simulink model "tracker"  (R2020a)
settings: Solver=VariableStepAuto  StartTime=0.0  StopTime=simulation_time  RelTol=1e-3
values from neighbouring files (symbols this model uses):
  costas_pll_arctan_nstage = 8    [tracker_hw_init.m]
  costas_pll_arctan_point = 16    [tracker_hw_init.m]
  costas_pll_arctan_width = 32    [tracker_hw_init.m]
  DDS_ch_pinc = fc.*(2^(DDS_phase_width)/fs)    [tracker_hw_init.m]
  fs = 120e6    (= 120000000)    [tracker_hw_init.m]
  normalized_EML_power_cordic_nstage = 11    [tracker_hw_init.m]
  normalized_EML_power_cordic_point = 32    [tracker_hw_init.m]
  normalized_EML_power_cordic_width = 32    [tracker_hw_init.m]
  ts = 1/fs    (= 8.33333333333e-09)    [tracker_hw_init.m]
undefined symbols (not defined in the file or in its folder): cacode, i
libraries: xbsIndex_r4 x1873
(part 1 of 14)
settings Model: Creator=User  LastModifiedBy=sysgen

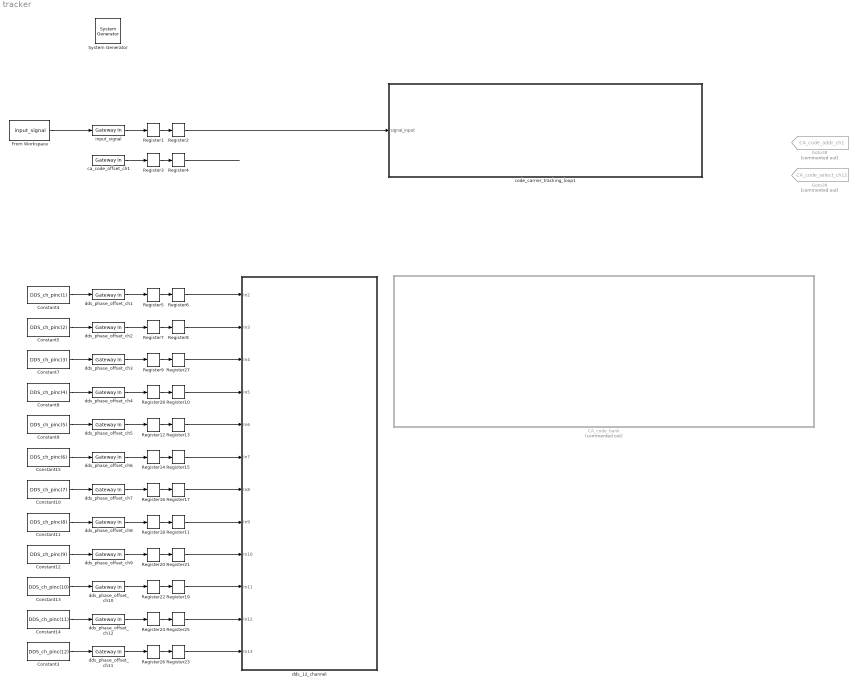
== system tracker ==
  " System Generator" : xbsIndex_r4/ System Generator  Tag=genX  xilinxfamily=zynquplus  part=xczu7ev  speed=-1-i  package=fbvb900  synthesis_tool=Vivado  clock_wrapper=Clock Enables  directory=./netlist  proj_type=Vivado  Synth_file=Vivado Synthesis Defaults  Impl_file=Vivado Implementation Defaults  testbench=off  simulink_period=ts  sysclk_period=ts*1e9  dcm_input_clock_period=10  incr_netlist=off  trim_vbits=Everywhere in SubSystem  dbl_ovrd=According to Block Masks  core_generation=According to Block Masks  run_coregen=off  deprecated_control=off  eval_field=0  block_type=sysgen
  CA_code_bank : Subsystem  Commented=on
  Constant10 : Constant  Value=DDS_ch_pinc(7)
  Constant11 : Constant  Value=DDS_ch_pinc(8)
  Constant12 : Constant  Value=DDS_ch_pinc(9)
  Constant13 : Constant  Value=DDS_ch_pinc(10)
  Constant14 : Constant  Value=DDS_ch_pinc(11)
  Constant15 : Constant  Value=DDS_ch_pinc(6)
  Constant3 : Constant  Value=DDS_ch_pinc(12)
  Constant4 : Constant  Value=DDS_ch_pinc(1)
  Constant5 : Constant  Value=DDS_ch_pinc(2)
  Constant7 : Constant  Value=DDS_ch_pinc(3)
  Constant8 : Constant  Value=DDS_ch_pinc(4)
  Constant9 : Constant  Value=DDS_ch_pinc(5)
  From Workspace : FromWorkspace  VariableName=input_signal  SampleTime=-1  OutputAfterFinalValue=Setting to zero
  Goto38 : Goto  Commented=on  GotoTag=CA_code_addr_ch1  TagVisibility=global
  Goto39 : Goto  Commented=on  GotoTag=CA_code_select_ch12  TagVisibility=global
  Register{1..28} (28 alike) : xbsIndex_r4/Register  init=0  rst=off  en=off  dbl_ovrd=off  block_type=register
  ca_code_offset_ch1 : xbsIndex_r4/Gateway In  gui_display_data_type=Fixed-point  arith_type=Unsigned  n_bits=DDS_phase_width  bin_pt=DDS_phase_width  preci_type=Single  exp_width=8  frac_width=24  rows=1  columns=1  quantization="Round  (unbiased: +/- Inf)"  overflow=Saturate  period=12*ts  UseAsADC=off  ADCChannel='1'  interface=None  automatic_assignment=on  address_offset=hex2dec('00')  intf_name=''  intf_description=''  default_value=0  timing_constraint=None  locs_specified=off  LOCs={}  io_standard={}  inherit_from_input=off  hdl_port=on  dbl_ovrd=off  block_type=gatewayin
  code_carrier_tracking_loop1 : Subsystem
  dds_12_channel : Subsystem
  dds_phase_offset_ch{1..12} (12 alike) : xbsIndex_r4/Gateway In  gui_display_data_type=Fixed-point  arith_type=Unsigned  n_bits=DDS_phase_width  bin_pt=DDS_phase_width  preci_type=Single  exp_width=8  frac_width=24  rows=1  columns=1  quantization="Round  (unbiased: +/- Inf)"  overflow=Saturate  period=ts  UseAsADC=off  ADCChannel='1'  interface=None  automatic_assignment=on  address_offset=hex2dec('00')  intf_name=''  intf_description=''  default_value=0  timing_constraint=None  locs_specified=off  LOCs={}  io_standard={}  inherit_from_input=off  hdl_port=on  dbl_ovrd=off  block_type=gatewayin
  input_signal : xbsIndex_r4/Gateway In  gui_display_data_type=Fixed-point  arith_type="Signed  (2's comp)"  n_bits=input_signal_width  bin_pt=input_signal_binary_point  preci_type=Single  exp_width=8  frac_width=24  rows=1  columns=1  quantization="Round  (unbiased: +/- Inf)"  overflow=Saturate  period=12*ts  UseAsADC=off  ADCChannel='1'  interface=None  automatic_assignment=on  address_offset=hex2dec('00')  intf_name=''  intf_description=''  default_value=0  timing_constraint=None  locs_specified=off  LOCs={}  io_standard={}  inherit_from_input=off  hdl_port=on  dbl_ovrd=off  block_type=gatewayin
  wires:
  dds_phase_offset_ch9/1 -> Register20/1
  Constant9/1 -> dds_phase_offset_ch5/1
  Constant4/1 -> dds_phase_offset_ch1/1
  Constant10/1 -> dds_phase_offset_ch7/1
  Constant11/1 -> dds_phase_offset_ch8/1
  Constant13/1 -> dds_phase_offset_ch10/1
  Constant3/1 -> dds_phase_offset_ch11/1
  dds_phase_offset_ch12/1 -> Register24/1
  Register22/1 -> Register19/1
  dds_phase_offset_ch6/1 -> Register14/1
  Register26/1 -> Register23/1
  dds_phase_offset_ch7/1 -> Register16/1
  Register20/1 -> Register21/1
  Constant12/1 -> dds_phase_offset_ch9/1
  Constant8/1 -> dds_phase_offset_ch4/1
  dds_phase_offset_ch11/1 -> Register26/1
  Constant5/1 -> dds_phase_offset_ch2/1
  Constant7/1 -> dds_phase_offset_ch3/1
  Constant15/1 -> dds_phase_offset_ch6/1
  dds_phase_offset_ch5/1 -> Register12/1
  Register24/1 -> Register25/1
  Constant14/1 -> dds_phase_offset_ch12/1
  dds_phase_offset_ch8/1 -> Register18/1
  Register5/1 -> Register6/1
  Register28/1 -> Register10/1
  dds_phase_offset_ch2/1 -> Register7/1
  Register18/1 -> Register11/1
  Register12/1 -> Register13/1
  dds_phase_offset_ch4/1 -> Register28/1
  Register16/1 -> Register17/1
  dds_phase_offset_ch3/1 -> Register9/1
  Register7/1 -> Register8/1
  Register9/1 -> Register27/1
  dds_phase_offset_ch1/1 -> Register5/1
  dds_phase_offset_ch10/1 -> Register22/1
  Register14/1 -> Register15/1
  Register6/1 -> dds_12_channel/1(In2)
  Register8/1 -> dds_12_channel/2(In3)
  Register27/1 -> dds_12_channel/3(In4)
  Register10/1 -> dds_12_channel/4(In5)
  Register13/1 -> dds_12_channel/5(In6)
  Register15/1 -> dds_12_channel/6(In7)
  Register17/1 -> dds_12_channel/7(In8)
  Register11/1 -> dds_12_channel/8(In9)
  Register21/1 -> dds_12_channel/9(In10)
  Register19/1 -> dds_12_channel/10(In11)
  Register25/1 -> dds_12_channel/11(In12)
  Register23/1 -> dds_12_channel/12(In13)
  input_signal/1 -> Register1/1
  Register1/1 -> Register2/1
  Register2/1 -> code_carrier_tracking_loop1/1(signal_input)
  From Workspace/1 -> input_signal/1
  Register4/1 -> ?
  ca_code_offset_ch1/1 -> Register3/1
  Register3/1 -> Register4/1

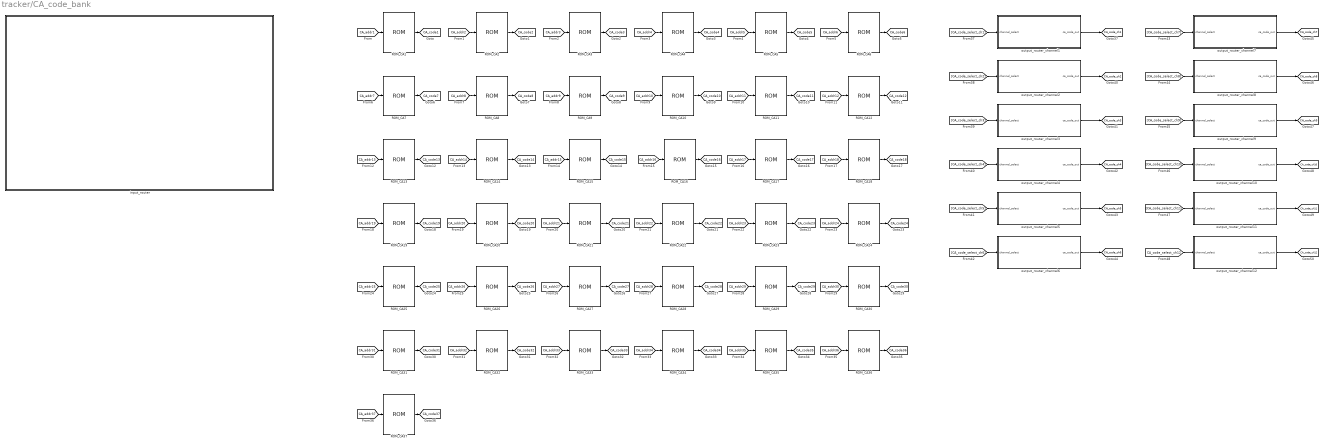
== system tracker/CA_code_bank ==
  ROM_CA1 : xbsIndex_r4/ROM  depth=1023  initVector=cacode(1,1)  distributed_mem=Distributed memory  rst=off  init_reg=0  en=off  latency=1  gui_display_data_type=Boolean  arith_type=Boolean  n_bits=16  bin_pt=14  preci_type=Single  exp_width=8  frac_width=24  optimize=Area  use_rpm=on  dbl_ovrd=off  simulation_type=fast_sim  block_type=sprom
  ROM_CA10 : xbsIndex_r4/ROM  depth=1023  initVector=cacode(10,1)  distributed_mem=Distributed memory  rst=off  init_reg=0  en=off  latency=1  gui_display_data_type=Boolean  arith_type=Boolean  n_bits=16  bin_pt=14  preci_type=Single  exp_width=8  frac_width=24  optimize=Area  use_rpm=on  dbl_ovrd=off  simulation_type=fast_sim  block_type=sprom
  ROM_CA11 : xbsIndex_r4/ROM  depth=1023  initVector=cacode(11,1)  distributed_mem=Distributed memory  rst=off  init_reg=0  en=off  latency=1  gui_display_data_type=Boolean  arith_type=Boolean  n_bits=16  bin_pt=14  preci_type=Single  exp_width=8  frac_width=24  optimize=Area  use_rpm=on  dbl_ovrd=off  simulation_type=fast_sim  block_type=sprom
  ROM_CA12 : xbsIndex_r4/ROM  depth=1023  initVector=cacode(12,1)  distributed_mem=Distributed memory  rst=off  init_reg=0  en=off  latency=1  gui_display_data_type=Boolean  arith_type=Boolean  n_bits=16  bin_pt=14  preci_type=Single  exp_width=8  frac_width=24  optimize=Area  use_rpm=on  dbl_ovrd=off  simulation_type=fast_sim  block_type=sprom
  ROM_CA13 : xbsIndex_r4/ROM  depth=1023  initVector=cacode(13,1)  distributed_mem=Distributed memory  rst=off  init_reg=0  en=off  latency=1  gui_display_data_type=Boolean  arith_type=Boolean  n_bits=16  bin_pt=14  preci_type=Single  exp_width=8  frac_width=24  optimize=Area  use_rpm=on  dbl_ovrd=off  simulation_type=fast_sim  block_type=sprom
  ROM_CA14 : xbsIndex_r4/ROM  depth=1023  initVector=cacode(14,1)  distributed_mem=Distributed memory  rst=off  init_reg=0  en=off  latency=1  gui_display_data_type=Boolean  arith_type=Boolean  n_bits=16  bin_pt=14  preci_type=Single  exp_width=8  frac_width=24  optimize=Area  use_rpm=on  dbl_ovrd=off  simulation_type=fast_sim  block_type=sprom
  ROM_CA15 : xbsIndex_r4/ROM  depth=1023  initVector=cacode(15,1)  distributed_mem=Distributed memory  rst=off  init_reg=0  en=off  latency=1  gui_display_data_type=Boolean  arith_type=Boolean  n_bits=16  bin_pt=14  preci_type=Single  exp_width=8  frac_width=24  optimize=Area  use_rpm=on  dbl_ovrd=off  simulation_type=fast_sim  block_type=sprom
  ROM_CA16 : xbsIndex_r4/ROM  depth=1023  initVector=cacode(16,1)  distributed_mem=Distributed memory  rst=off  init_reg=0  en=off  latency=1  gui_display_data_type=Boolean  arith_type=Boolean  n_bits=16  bin_pt=14  preci_type=Single  exp_width=8  frac_width=24  optimize=Area  use_rpm=on  dbl_ovrd=off  simulation_type=fast_sim  block_type=sprom
  ROM_CA17 : xbsIndex_r4/ROM  depth=1023  initVector=cacode(17,1)  distributed_mem=Distributed memory  rst=off  init_reg=0  en=off  latency=1  gui_display_data_type=Boolean  arith_type=Boolean  n_bits=16  bin_pt=14  preci_type=Single  exp_width=8  frac_width=24  optimize=Area  use_rpm=on  dbl_ovrd=off  simulation_type=fast_sim  block_type=sprom
  ROM_CA18 : xbsIndex_r4/ROM  depth=1023  initVector=cacode(18,1)  distributed_mem=Distributed memory  rst=off  init_reg=0  en=off  latency=1  gui_display_data_type=Boolean  arith_type=Boolean  n_bits=16  bin_pt=14  preci_type=Single  exp_width=8  frac_width=24  optimize=Area  use_rpm=on  dbl_ovrd=off  simulation_type=fast_sim  block_type=sprom
  ROM_CA19 : xbsIndex_r4/ROM  depth=1023  initVector=cacode(19,1)  distributed_mem=Distributed memory  rst=off  init_reg=0  en=off  latency=1  gui_display_data_type=Boolean  arith_type=Boolean  n_bits=16  bin_pt=14  preci_type=Single  exp_width=8  frac_width=24  optimize=Area  use_rpm=on  dbl_ovrd=off  simulation_type=fast_sim  block_type=sprom
  ROM_CA2 : xbsIndex_r4/ROM  depth=1023  initVector=cacode(2,1)  distributed_mem=Distributed memory  rst=off  init_reg=0  en=off  latency=1  gui_display_data_type=Boolean  arith_type=Boolean  n_bits=16  bin_pt=14  preci_type=Single  exp_width=8  frac_width=24  optimize=Area  use_rpm=on  dbl_ovrd=off  simulation_type=fast_sim  block_type=sprom
  ROM_CA20 : xbsIndex_r4/ROM  depth=1023  initVector=cacode(20,1)  distributed_mem=Distributed memory  rst=off  init_reg=0  en=off  latency=1  gui_display_data_type=Boolean  arith_type=Boolean  n_bits=16  bin_pt=14  preci_type=Single  exp_width=8  frac_width=24  optimize=Area  use_rpm=on  dbl_ovrd=off  simulation_type=fast_sim  block_type=sprom
  ROM_CA21 : xbsIndex_r4/ROM  depth=1023  initVector=cacode(21,1)  distributed_mem=Distributed memory  rst=off  init_reg=0  en=off  latency=1  gui_display_data_type=Boolean  arith_type=Boolean  n_bits=16  bin_pt=14  preci_type=Single  exp_width=8  frac_width=24  optimize=Area  use_rpm=on  dbl_ovrd=off  simulation_type=fast_sim  block_type=sprom
  ROM_CA22 : xbsIndex_r4/ROM  depth=1023  initVector=cacode(22,1)  distributed_mem=Distributed memory  rst=off  init_reg=0  en=off  latency=1  gui_display_data_type=Boolean  arith_type=Boolean  n_bits=16  bin_pt=14  preci_type=Single  exp_width=8  frac_width=24  optimize=Area  use_rpm=on  dbl_ovrd=off  simulation_type=fast_sim  block_type=sprom
  ROM_CA23 : xbsIndex_r4/ROM  depth=1023  initVector=cacode(23,1)  distributed_mem=Distributed memory  rst=off  init_reg=0  en=off  latency=1  gui_display_data_type=Boolean  arith_type=Boolean  n_bits=16  bin_pt=14  preci_type=Single  exp_width=8  frac_width=24  optimize=Area  use_rpm=on  dbl_ovrd=off  simulation_type=fast_sim  block_type=sprom
  ROM_CA24 : xbsIndex_r4/ROM  depth=1023  initVector=cacode(24,1)  distributed_mem=Distributed memory  rst=off  init_reg=0  en=off  latency=1  gui_display_data_type=Boolean  arith_type=Boolean  n_bits=16  bin_pt=14  preci_type=Single  exp_width=8  frac_width=24  optimize=Area  use_rpm=on  dbl_ovrd=off  simulation_type=fast_sim  block_type=sprom
  ROM_CA25 : xbsIndex_r4/ROM  depth=1023  initVector=cacode(25,1)  distributed_mem=Distributed memory  rst=off  init_reg=0  en=off  latency=1  gui_display_data_type=Boolean  arith_type=Boolean  n_bits=16  bin_pt=14  preci_type=Single  exp_width=8  frac_width=24  optimize=Area  use_rpm=on  dbl_ovrd=off  simulation_type=fast_sim  block_type=sprom
  ROM_CA26 : xbsIndex_r4/ROM  depth=1023  initVector=cacode(26,1)  distributed_mem=Distributed memory  rst=off  init_reg=0  en=off  latency=1  gui_display_data_type=Boolean  arith_type=Boolean  n_bits=16  bin_pt=14  preci_type=Single  exp_width=8  frac_width=24  optimize=Area  use_rpm=on  dbl_ovrd=off  simulation_type=fast_sim  block_type=sprom
  ROM_CA27 : xbsIndex_r4/ROM  depth=1023  initVector=cacode(27,1)  distributed_mem=Distributed memory  rst=off  init_reg=0  en=off  latency=1  gui_display_data_type=Boolean  arith_type=Boolean  n_bits=16  bin_pt=14  preci_type=Single  exp_width=8  frac_width=24  optimize=Area  use_rpm=on  dbl_ovrd=off  simulation_type=fast_sim  block_type=sprom
  ROM_CA28 : xbsIndex_r4/ROM  depth=1023  initVector=cacode(28,1)  distributed_mem=Distributed memory  rst=off  init_reg=0  en=off  latency=1  gui_display_data_type=Boolean  arith_type=Boolean  n_bits=16  bin_pt=14  preci_type=Single  exp_width=8  frac_width=24  optimize=Area  use_rpm=on  dbl_ovrd=off  simulation_type=fast_sim  block_type=sprom
  ROM_CA29 : xbsIndex_r4/ROM  depth=1023  initVector=cacode(29,1)  distributed_mem=Distributed memory  rst=off  init_reg=0  en=off  latency=1  gui_display_data_type=Boolean  arith_type=Boolean  n_bits=16  bin_pt=14  preci_type=Single  exp_width=8  frac_width=24  optimize=Area  use_rpm=on  dbl_ovrd=off  simulation_type=fast_sim  block_type=sprom
  ROM_CA3 : xbsIndex_r4/ROM  depth=1023  initVector=cacode(3,1)  distributed_mem=Distributed memory  rst=off  init_reg=0  en=off  latency=1  gui_display_data_type=Boolean  arith_type=Boolean  n_bits=16  bin_pt=14  preci_type=Single  exp_width=8  frac_width=24  optimize=Area  use_rpm=on  dbl_ovrd=off  simulation_type=fast_sim  block_type=sprom
  ROM_CA30 : xbsIndex_r4/ROM  depth=1023  initVector=cacode(30,1)  distributed_mem=Distributed memory  rst=off  init_reg=0  en=off  latency=1  gui_display_data_type=Boolean  arith_type=Boolean  n_bits=16  bin_pt=14  preci_type=Single  exp_width=8  frac_width=24  optimize=Area  use_rpm=on  dbl_ovrd=off  simulation_type=fast_sim  block_type=sprom
  ROM_CA31 : xbsIndex_r4/ROM  depth=1023  initVector=cacode(31,1)  distributed_mem=Distributed memory  rst=off  init_reg=0  en=off  latency=1  gui_display_data_type=Boolean  arith_type=Boolean  n_bits=16  bin_pt=14  preci_type=Single  exp_width=8  frac_width=24  optimize=Area  use_rpm=on  dbl_ovrd=off  simulation_type=fast_sim  block_type=sprom
  ROM_CA32 : xbsIndex_r4/ROM  depth=1023  initVector=cacode(32,1)  distributed_mem=Distributed memory  rst=off  init_reg=0  en=off  latency=1  gui_display_data_type=Boolean  arith_type=Boolean  n_bits=16  bin_pt=14  preci_type=Single  exp_width=8  frac_width=24  optimize=Area  use_rpm=on  dbl_ovrd=off  simulation_type=fast_sim  block_type=sprom
  ROM_CA33 : xbsIndex_r4/ROM  depth=1023  initVector=cacode(33,1)  distributed_mem=Distributed memory  rst=off  init_reg=0  en=off  latency=1  gui_display_data_type=Boolean  arith_type=Boolean  n_bits=16  bin_pt=14  preci_type=Single  exp_width=8  frac_width=24  optimize=Area  use_rpm=on  dbl_ovrd=off  simulation_type=fast_sim  block_type=sprom
  ROM_CA34 : xbsIndex_r4/ROM  depth=1023  initVector=cacode(34,1)  distributed_mem=Distributed memory  rst=off  init_reg=0  en=off  latency=1  gui_display_data_type=Boolean  arith_type=Boolean  n_bits=16  bin_pt=14  preci_type=Single  exp_width=8  frac_width=24  optimize=Area  use_rpm=on  dbl_ovrd=off  simulation_type=fast_sim  block_type=sprom
  ROM_CA35 : xbsIndex_r4/ROM  depth=1023  initVector=cacode(35,1)  distributed_mem=Distributed memory  rst=off  init_reg=0  en=off  latency=1  gui_display_data_type=Boolean  arith_type=Boolean  n_bits=16  bin_pt=14  preci_type=Single  exp_width=8  frac_width=24  optimize=Area  use_rpm=on  dbl_ovrd=off  simulation_type=fast_sim  block_type=sprom
  ROM_CA36 : xbsIndex_r4/ROM  depth=1023  initVector=cacode(36,1)  distributed_mem=Distributed memory  rst=off  init_reg=0  en=off  latency=1  gui_display_data_type=Boolean  arith_type=Boolean  n_bits=16  bin_pt=14  preci_type=Single  exp_width=8  frac_width=24  optimize=Area  use_rpm=on  dbl_ovrd=off  simulation_type=fast_sim  block_type=sprom
  ROM_CA37 : xbsIndex_r4/ROM  depth=1023  initVector=cacode(37,1)  distributed_mem=Distributed memory  rst=off  init_reg=0  en=off  latency=1  gui_display_data_type=Boolean  arith_type=Boolean  n_bits=16  bin_pt=14  preci_type=Single  exp_width=8  frac_width=24  optimize=Area  use_rpm=on  dbl_ovrd=off  simulation_type=fast_sim  block_type=sprom
  ROM_CA4 : xbsIndex_r4/ROM  depth=1023  initVector=cacode(4,1)  distributed_mem=Distributed memory  rst=off  init_reg=0  en=off  latency=1  gui_display_data_type=Boolean  arith_type=Boolean  n_bits=16  bin_pt=14  preci_type=Single  exp_width=8  frac_width=24  optimize=Area  use_rpm=on  dbl_ovrd=off  simulation_type=fast_sim  block_type=sprom
  ROM_CA5 : xbsIndex_r4/ROM  depth=1023  initVector=cacode(5,1)  distributed_mem=Distributed memory  rst=off  init_reg=0  en=off  latency=1  gui_display_data_type=Boolean  arith_type=Boolean  n_bits=16  bin_pt=14  preci_type=Single  exp_width=8  frac_width=24  optimize=Area  use_rpm=on  dbl_ovrd=off  simulation_type=fast_sim  block_type=sprom
  ROM_CA6 : xbsIndex_r4/ROM  depth=1023  initVector=cacode(6,1)  distributed_mem=Distributed memory  rst=off  init_reg=0  en=off  latency=1  gui_display_data_type=Boolean  arith_type=Boolean  n_bits=16  bin_pt=14  preci_type=Single  exp_width=8  frac_width=24  optimize=Area  use_rpm=on  dbl_ovrd=off  simulation_type=fast_sim  block_type=sprom
  ROM_CA7 : xbsIndex_r4/ROM  depth=1023  initVector=cacode(7,1)  distributed_mem=Distributed memory  rst=off  init_reg=0  en=off  latency=1  gui_display_data_type=Boolean  arith_type=Boolean  n_bits=16  bin_pt=14  preci_type=Single  exp_width=8  frac_width=24  optimize=Area  use_rpm=on  dbl_ovrd=off  simulation_type=fast_sim  block_type=sprom
  ROM_CA8 : xbsIndex_r4/ROM  depth=1023  initVector=cacode(8,1)  distributed_mem=Distributed memory  rst=off  init_reg=0  en=off  latency=1  gui_display_data_type=Boolean  arith_type=Boolean  n_bits=16  bin_pt=14  preci_type=Single  exp_width=8  frac_width=24  optimize=Area  use_rpm=on  dbl_ovrd=off  simulation_type=fast_sim  block_type=sprom
  ROM_CA9 : xbsIndex_r4/ROM  depth=1023  initVector=cacode(9,1)  distributed_mem=Distributed memory  rst=off  init_reg=0  en=off  latency=1  gui_display_data_type=Boolean  arith_type=Boolean  n_bits=16  bin_pt=14  preci_type=Single  exp_width=8  frac_width=24  optimize=Area  use_rpm=on  dbl_ovrd=off  simulation_type=fast_sim  block_type=sprom
  input_router : Subsystem
  output_router_channel1 : Subsystem
  output_router_channel10 : Subsystem
  output_router_channel11 : Subsystem
  output_router_channel12 : Subsystem
  output_router_channel2 : Subsystem
  output_router_channel3 : Subsystem
  output_router_channel4 : Subsystem
  output_router_channel5 : Subsystem
  output_router_channel6 : Subsystem
  output_router_channel7 : Subsystem
  output_router_channel8 : Subsystem
  output_router_channel9 : Subsystem
  tag scope: CA_code10=global, CA_code11=global, CA_code12=global, CA_code13=global, CA_code14=global, CA_code15=global, CA_code16=global, CA_code17=global, CA_code18=global, CA_code19=global, CA_code1=global, CA_code20=global, CA_code21=global, CA_code22=global, CA_code23=global, CA_code24=global, CA_code25=global, CA_code26=global, CA_code27=global, CA_code28=global, CA_code29=global, CA_code2=global, CA_code30=global, CA_code31=global, CA_code32=global, CA_code33=global, CA_code34=global, CA_code35=global, CA_code36=global, CA_code37=global, CA_code3=global, CA_code4=global, CA_code5=global, CA_code6=global, CA_code7=global, CA_code8=global, CA_code9=global, CA_code_ch10=global, CA_code_ch11=global, CA_code_ch12=global, CA_code_ch1=global, CA_code_ch2=global, CA_code_ch3=global, CA_code_ch4=global, CA_code_ch5=global, CA_code_ch6=global, CA_code_ch7=global, CA_code_ch8=global, CA_code_ch9=global
  wires:
  ROM_CA1/1 -> [CA_code1]
  ROM_CA2/1 -> [CA_code2]
  ROM_CA3/1 -> [CA_code3]
  ROM_CA4/1 -> [CA_code4]
  ROM_CA5/1 -> [CA_code5]
  ROM_CA6/1 -> [CA_code6]
  ROM_CA7/1 -> [CA_code7]
  ROM_CA8/1 -> [CA_code8]
  ROM_CA9/1 -> [CA_code9]
  ROM_CA10/1 -> [CA_code10]
  ROM_CA11/1 -> [CA_code11]
  ROM_CA12/1 -> [CA_code12]
  ROM_CA13/1 -> [CA_code13]
  ROM_CA14/1 -> [CA_code14]
  ROM_CA15/1 -> [CA_code15]
  ROM_CA16/1 -> [CA_code16]
  ROM_CA17/1 -> [CA_code17]
  ROM_CA18/1 -> [CA_code18]
  ROM_CA19/1 -> [CA_code19]
  [CA_addr1] -> ROM_CA1/1
  [CA_addr2] -> ROM_CA2/1
  [CA_addr3] -> ROM_CA3/1
  [CA_addr4] -> ROM_CA4/1
  [CA_addr5] -> ROM_CA5/1
  [CA_addr6] -> ROM_CA6/1
  [CA_addr7] -> ROM_CA7/1
  [CA_addr8] -> ROM_CA8/1
  [CA_addr9] -> ROM_CA9/1
  [CA_addr10] -> ROM_CA10/1
  [CA_addr11] -> ROM_CA11/1
  [CA_addr12] -> ROM_CA12/1
  [CA_addr13] -> ROM_CA13/1
  [CA_addr14] -> ROM_CA14/1
  [CA_addr15] -> ROM_CA15/1
  [CA_addr16] -> ROM_CA16/1
  [CA_addr17] -> ROM_CA17/1
  [CA_addr18] -> ROM_CA18/1
  [CA_addr19] -> ROM_CA19/1
  [CA_addr20] -> ROM_CA20/1
  ROM_CA20/1 -> [CA_code20]
  [CA_addr21] -> ROM_CA21/1
  ROM_CA21/1 -> [CA_code21]
  [CA_addr22] -> ROM_CA22/1
  ROM_CA22/1 -> [CA_code22]
  [CA_addr23] -> ROM_CA23/1
  ROM_CA23/1 -> [CA_code23]
  [CA_addr24] -> ROM_CA24/1
  ROM_CA24/1 -> [CA_code24]
  [CA_addr25] -> ROM_CA25/1
  ROM_CA25/1 -> [CA_code25]
  [CA_addr26] -> ROM_CA26/1
  ROM_CA26/1 -> [CA_code26]
  [CA_addr27] -> ROM_CA27/1
  ROM_CA27/1 -> [CA_code27]
  ROM_CA28/1 -> [CA_code28]
  [CA_addr28] -> ROM_CA28/1
  ROM_CA29/1 -> [CA_code29]
  [CA_addr29] -> ROM_CA29/1
  [CA_addr30] -> ROM_CA30/1
  ROM_CA30/1 -> [CA_code30]
  [CA_addr31] -> ROM_CA31/1
  ROM_CA31/1 -> [CA_code31]
  [CA_addr32] -> ROM_CA32/1
  ROM_CA32/1 -> [CA_code32]
  [CA_addr33] -> ROM_CA33/1
  ROM_CA33/1 -> [CA_code33]
  [CA_addr34] -> ROM_CA34/1
  ROM_CA34/1 -> [CA_code34]
  [CA_addr35] -> ROM_CA35/1
  ROM_CA35/1 -> [CA_code35]
  [CA_addr36] -> ROM_CA36/1
  ROM_CA36/1 -> [CA_code36]
  ROM_CA37/1 -> [CA_code37]
  [CA_addr37] -> ROM_CA37/1
  output_router_channel1/1(ca_code_out) -> [CA_code_ch1]
  [CA_code_select_ch1] -> output_router_channel1/1(channel_select)
  [CA_code_select_ch2] -> output_router_channel2/1(channel_select)
  output_router_channel2/1(ca_code_out) -> [CA_code_ch2]
  output_router_channel3/1(ca_code_out) -> [CA_code_ch3]
  [CA_code_select_ch3] -> output_router_channel3/1(channel_select)
  [CA_code_select_ch6] -> output_router_channel6/1(channel_select)
  output_router_channel6/1(ca_code_out) -> [CA_code_ch6]
  output_router_channel5/1(ca_code_out) -> [CA_code_ch5]
  [CA_code_select_ch5] -> output_router_channel5/1(channel_select)
  [CA_code_select_ch4] -> output_router_channel4/1(channel_select)
  output_router_channel4/1(ca_code_out) -> [CA_code_ch4]
  output_router_channel10/1(ca_code_out) -> [CA_code_ch10]
  [CA_code_select_ch10] -> output_router_channel10/1(channel_select)
  [CA_code_select_ch11] -> output_router_channel11/1(channel_select)
  output_router_channel11/1(ca_code_out) -> [CA_code_ch11]
  output_router_channel12/1(ca_code_out) -> [CA_code_ch12]
  [CA_code_select_ch12] -> output_router_channel12/1(channel_select)
  [CA_code_select_ch9] -> output_router_channel9/1(channel_select)
  output_router_channel9/1(ca_code_out) -> [CA_code_ch9]
  output_router_channel8/1(ca_code_out) -> [CA_code_ch8]
  [CA_code_select_ch8] -> output_router_channel8/1(channel_select)
  [CA_code_select_ch7] -> output_router_channel7/1(channel_select)
  output_router_channel7/1(ca_code_out) -> [CA_code_ch7]

== system tracker/code_carrier_tracking_loop1 ==
  signal_input : Inport
  From49 : From  Commented=on  GotoTag=CA_code_ch1
  Mult_i : xbsIndex_r4/Mult  precision=Full  arith_type="Signed  (2's comp)"  n_bits=16  bin_pt=14  quantization=Truncate  overflow=Wrap  en=off  latency=3  use_behavioral_HDL=off  opt=Speed  use_embedded=on  optimum_pipeline=off  pipeline=on  dbl_ovrd=off  use_rpm=on  placement_style=Triangular  block_type=mult
  Mult_q : xbsIndex_r4/Mult  precision=Full  arith_type="Signed  (2's comp)"  n_bits=16  bin_pt=14  quantization=Truncate  overflow=Wrap  en=off  latency=3  use_behavioral_HDL=off  opt=Speed  use_embedded=on  optimum_pipeline=off  pipeline=on  dbl_ovrd=off  use_rpm=on  placement_style=Triangular  block_type=mult
  Register : xbsIndex_r4/Register  Commented=on  init=0  rst=off  en=off  dbl_ovrd=off  block_type=register
  Register29 : xbsIndex_r4/Register  Commented=on  init=0  rst=off  en=off  dbl_ovrd=off  block_type=register
  carrier_loop_discriminator : Subsystem  Commented=on
  code_loop_discriminator : Subsystem  Commented=on
  integration_and_dump_ie : Subsystem  Commented=on
  integration_and_dump_il : Subsystem  Commented=on
  integration_and_dump_ip : Subsystem  Commented=on
  integration_and_dump_qe : Subsystem  Commented=on
  integration_and_dump_ql : Subsystem  Commented=on
  integration_and_dump_qp : Subsystem  Commented=on
  wires:
  Register/1 -> integration_and_dump_ip/2(add_sub), integration_and_dump_qp/2(add_sub), Register29/1
  [cos_ch1] -> Mult_q/2
  Mult_i/1 -> integration_and_dump_il/1(data_in), integration_and_dump_ip/1(data_in), integration_and_dump_ie/1(data_in)
  signal_input/1 -> Mult_q/1, Mult_i/2
  From49/1 -> integration_and_dump_ie/2(add_sub), integration_and_dump_qe/2(add_sub), Register/1
  [sin_ch1] -> Mult_i/1
  Mult_q/1 -> integration_and_dump_qe/1(data_in), integration_and_dump_qp/1(data_in), integration_and_dump_ql/1(data_in)
  Register29/1 -> integration_and_dump_il/2(add_sub), integration_and_dump_ql/2(add_sub)
  integration_and_dump_ie/1(data_out) -> code_loop_discriminator/1(Ies)
  integration_and_dump_il/1(data_out) -> code_loop_discriminator/2(Ils)
  integration_and_dump_qe/1(data_out) -> code_loop_discriminator/3(Qes)
  integration_and_dump_ql/1(data_out) -> code_loop_discriminator/4(Qls)
  integration_and_dump_ip/1(data_out) -> carrier_loop_discriminator/1(Ips)
  integration_and_dump_qp/1(data_out) -> carrier_loop_discriminator/2(Qps)

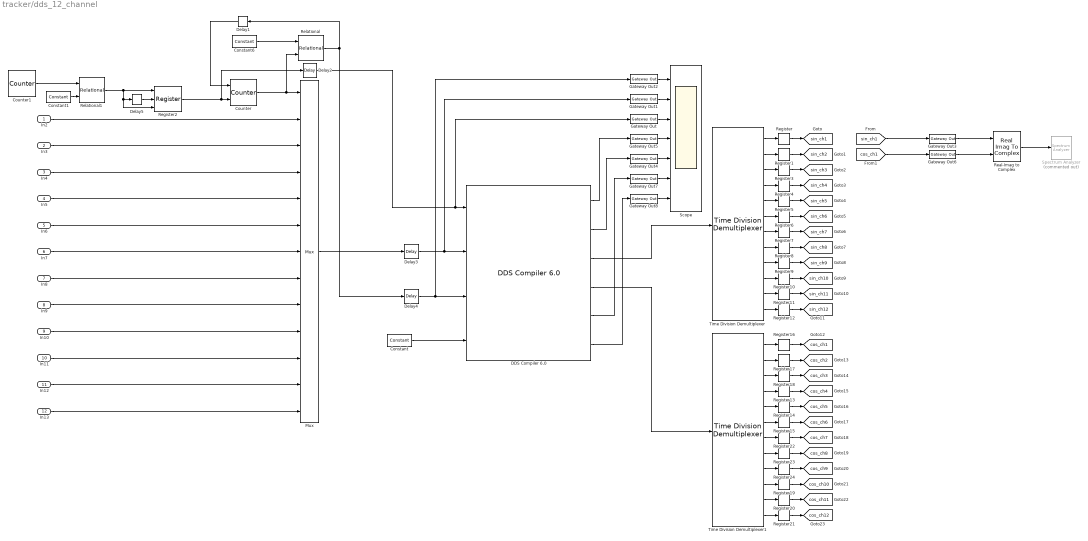
== system tracker/dds_12_channel ==
  In2 : Inport
  In3 : Inport  Port=2
  In4 : Inport  Port=3
  In5 : Inport  Port=4
  In6 : Inport  Port=5
  In7 : Inport  Port=6
  In8 : Inport  Port=7
  In9 : Inport  Port=8
  In10 : Inport  Port=9
  In11 : Inport  Port=10
  In12 : Inport  Port=11
  In13 : Inport  Port=12
  Constant : xbsIndex_r4/Constant  const=1.0  gui_display_data_type=Boolean  arith_type=Boolean  n_bits=16  bin_pt=14  preci_type=Single  exp_width=8  frac_width=24  explicit_period=on  period=ts  equ=P=C  opselect=C  inp2=PCIN>>17  opr=+  inp1=P  carry=CIN  dbl_ovrd=off  block_type=constant
  Constant1 : xbsIndex_r4/Constant  const=1000  gui_display_data_type=Fixed-point  arith_type=Unsigned  n_bits=10  bin_pt=0  preci_type=Single  exp_width=8  frac_width=24  explicit_period=off  period=1  equ=P=C  opselect=C  inp2=PCIN>>17  opr=+  inp1=P  carry=CIN  dbl_ovrd=off  block_type=constant
  Constant6 : xbsIndex_r4/Constant  const=11  gui_display_data_type=Fixed-point  arith_type=Unsigned  n_bits=4  bin_pt=0  preci_type=Single  exp_width=8  frac_width=24  explicit_period=off  period=1  equ=P=C  opselect=C  inp2=PCIN>>17  opr=+  inp1=P  carry=CIN  dbl_ovrd=off  block_type=constant
  Counter : xbsIndex_r4/Counter  cnt_type=Count Limited  cnt_to=11  operation=Up  start_count=0  cnt_by_val=1  arith_type=Unsigned  n_bits=4  bin_pt=0  load_pin=off  rst=on  en=on  explicit_period=on  period=ts  use_behavioral_HDL=off  implementation=Fabric  dbl_ovrd=off  block_type=counter
  Counter1 : xbsIndex_r4/Counter  cnt_type=Free Running  cnt_to=Inf  operation=Up  start_count=0  cnt_by_val=1  arith_type=Unsigned  n_bits=10  bin_pt=0  load_pin=off  rst=off  en=off  explicit_period=on  period=ts  use_behavioral_HDL=off  implementation=Fabric  dbl_ovrd=off  block_type=counter
  "DDS Compiler 6.0 " : xbsIndex_r4/DDS Compiler 6.0   partspresent=Phase_Generator_and_SIN_COS_LUT  dds_clock_rate=fs*1e-6  channels=12  mode_of_operation=Standard  modulus=9  parameter_entry=Hardware_Parameters  spurious_free_dynamic_range=70.00000000  frequency_resolution=0.40000000  noise_shaping=None  phase_width=DDS_phase_width  output_width=DDS_signal_width  output_selection=Sine_and_Cosine  negative_sine=off  negative_cosine=off  amplitude_mode=Full_Range  memory_type=Auto  optimization_goal=Auto  dsp48_use=Minimal  resync=off  latency_configuration=Auto  latency=1  has_phase_out=off  has_aclken=off  has_aresetn=off  explicit_period=off  period=1  data_has_tlast=Not_Required  has_tready=on  s_phase_has_tuser=Not_Required  m_data_has_tuser=Not_Required  m_phase_has_tuser=Not_Required  s_phase_tuser_width=1  output_form=Twos_Complement  s_config_sync_mode=On_Vector  phase_increment=Programmable  output_frequency1=0  output_frequency2=0  output_frequency3=0  output_frequency4=0  output_frequency5=0  output_frequency6=0  output_frequency7=0  output_frequency8=0  output_frequency9=0  output_frequency10=0  output_frequency11=0  output_frequency12=0  output_frequency13=0  output_frequency14=0  output_frequency15=0  output_frequency16=0  pinc1='1101000110110111'  pinc2='1101000111110111'  pinc3='1101010110110111'  pinc4='1101100110110111'  pinc5='1101000110110111'  pinc6='1101000110110111'  pinc7='1101000110010111'  pinc8='1101000111110111'  pinc9='1101000110110111'  pinc10='1101000110110111'  pinc11='1101010110110111'  pinc12='1101000110110111'  pinc13='0'  pinc14='0'  pinc15='0'  pinc16='0'  phase_offset=None  phase_offset_angles1=0  phase_offset_angles2=0  phase_offset_angles3=0  phase_offset_angles4=0  phase_offset_angles5=0  phase_offset_angles6=0  phase_offset_angles7=0  phase_offset_angles8=0  phase_offset_angles9=0  phase_offset_angles10=0  phase_offset_angles11=0  phase_offset_angles12=0  phase_offset_angles13=0  phase_offset_angles14=0  phase_offset_angles15=0  phase_offset_angles16=0  poff1='0'  poff2='0'  poff3='0'  poff4='0'  poff5='0'  poff6='0'  poff7='0'  poff8='0'  poff9='0'  poff10='0'  poff11='0'  poff12='0'  poff13='0'  poff14='0'  poff15='0'  poff16='0'  trim_axipin_name=on  simulation_type=hybrid_sim  simulation_model=sysgen:xddsv6_0_cmodel  data_path_portlist={ 's_axis_config_tdata_poff', 's_axis_config_tdata_chan0_poff', 's_axis_config_tdata_pinc', 's_axis_config_tdata_chan0_pinc', 's_axis_phase_tdata_resync', 's_axis_phase_tdata_chan0_resync', 's_axis_phase_tdata_poff', 's_axis_phase_tdata_chan0_poff', 's_axis_phase_tdata_pinc', 's_axis_phase_tdata_chan0_pinc', 's_axis_phase_tdata_phase_in', 'm_axis_data_tdata_sine', 'm_axis_data_tdata_chan0_sine', 'm_axis_data_tdata_cosine', 'm_axis_data_tdata_chan0_cosine', 'm_axis_phase_tdata_phase_out', 'm_axis_phase_tdata_chan0_phase_out'}  por_mode=false  gui_behaviour=Sysgen  ip_name=DDS Compiler  ip_version=6.0  dsptool_ready=true  wrapper_available=true  port_translation_map={ 'aclken' => 'en', 'aresetn' => 'rst' }  ipcore_usecache=true  ipcore_useipmodelcache=true  ipcore_xco_need_fpga_part=true  ipcore_verbose=false  block_type=dds_compiler_v6_0
  Delay1 : xbsIndex_r4/Delay  rst=off  infoeditControl=Selection of Reset will increase slice count due to use of real FFs and instead of SRLs  en=off  latency=5  reg_retiming=off  dbl_ovrd=off  block_type=delay
  Delay2 : xbsIndex_r4/Delay  rst=off  infoeditControl=Selection of Reset will increase slice count due to use of real FFs and instead of SRLs  en=off  latency=2  reg_retiming=off  dbl_ovrd=off  block_type=delay
  Delay3 : xbsIndex_r4/Delay  rst=off  infoeditControl=Selection of Reset will increase slice count due to use of real FFs and instead of SRLs  en=off  latency=1  reg_retiming=off  dbl_ovrd=off  block_type=delay
  Delay4 : xbsIndex_r4/Delay  rst=off  infoeditControl=Selection of Reset will increase slice count due to use of real FFs and instead of SRLs  en=off  latency=1  reg_retiming=off  dbl_ovrd=off  block_type=delay
  Delay5 : xbsIndex_r4/Delay  rst=off  infoeditControl=Selection of Reset will increase slice count due to use of real FFs and instead of SRLs  en=off  latency=12  reg_retiming=off  dbl_ovrd=off  block_type=delay
  Gateway Out{,1..8} (9 alike) : xbsIndex_r4/Gateway Out  inherit_from_input=off  hdl_port=off  rows=1  columns=1  UseAsDAC=off  DACChannel='1'  interface=None  automatic_assignment=on  address_offset=hex2dec('00')  intf_name=''  intf_description=''  timing_constraint=None  locs_specified=off  LOCs={}  io_standard={}  block_type=gatewayout
  Mux : xbsIndex_r4/Mux  inputs=12  en=off  latency=1  precision=Full  arith_type=Unsigned  n_bits=16  bin_pt=14  quantization=Truncate  overflow=Wrap  dbl_ovrd=off  block_type=mux
  Real-Imag to Complex : RealImagToComplex
  Register{,1,3..24} (24 alike) : xbsIndex_r4/Register  init=0  rst=off  en=off  dbl_ovrd=off  block_type=register
  Register2 : xbsIndex_r4/Register  init=0  rst=on  en=on  dbl_ovrd=off  block_type=register
  Relational : xbsIndex_r4/Relational  mode=a=b  op_type=Bool  en=off  latency=1  dbl_ovrd=off  block_type=relational
  Relational1 : xbsIndex_r4/Relational  mode=a=b  op_type=Bool  en=off  latency=1  dbl_ovrd=off  block_type=relational
  Scope : Scope  NumInputPorts=7
  Spectrum Analyzer : SpectrumAnalyzer  Commented=on
  Time Division Demultiplexer : xbsIndex_r4/Time Division Demultiplexer  frame_pattern=ones(1,12)  impl_style=Multiple Channel  vin=off  explicit_period=off  dbl_ovrd=off  period=1  block_type=tdd
      settings: infoedit=Samples presented at the input are selected and down-sampled according to the frame sampling pattern specified. The sampled input is presented either as a single or multiple channel at the output.
  Time Division Demultiplexer1 : xbsIndex_r4/Time Division Demultiplexer  frame_pattern=ones(1,12)  impl_style=Multiple Channel  vin=off  explicit_period=off  dbl_ovrd=off  period=1  block_type=tdd
      settings: infoedit=Samples presented at the input are selected and down-sampled according to the frame sampling pattern specified. The sampled input is presented either as a single or multiple channel at the output.
  tag scope: cos_ch10=global, cos_ch11=global, cos_ch12=global, cos_ch1=global, cos_ch2=global, cos_ch3=global, cos_ch4=global, cos_ch5=global, cos_ch6=global, cos_ch7=global, cos_ch8=global, cos_ch9=global, sin_ch10=global, sin_ch11=global, sin_ch12=global, sin_ch1=global, sin_ch2=global, sin_ch3=global, sin_ch4=global, sin_ch5=global, sin_ch6=global, sin_ch7=global, sin_ch8=global, sin_ch9=global
  wires:
  Register2/1 -> Delay2/1, Counter/2
  Mux/1 -> Delay3/1
  Counter/1 -> Relational/2, Mux/1
  Constant6/1 -> Relational/1
  Relational/1 -> Delay1/1, Delay4/1
  Delay3/1 -> Gateway Out1/1, "DDS Compiler 6.0 "/2
  Relational1/1 -> Delay5/1, Register2/3, Register2/1
  Delay1/1 -> Counter/1
  Delay5/1 -> Register2/2
  Delay2/1 -> Gateway Out/1, "DDS Compiler 6.0 "/1
  Delay4/1 -> Gateway Out2/1, "DDS Compiler 6.0 "/3
  In7/1 -> Mux/7
  In11/1 -> Mux/11
  In5/1 -> Mux/5
  In6/1 -> Mux/6
  In4/1 -> Mux/4
  In3/1 -> Mux/3
  In13/1 -> Mux/13
  In8/1 -> Mux/8
  In2/1 -> Mux/2
  In10/1 -> Mux/10
  In9/1 -> Mux/9
  In12/1 -> Mux/12
  Gateway Out2/1 -> Scope/1
  Gateway Out1/1 -> Scope/2
  Gateway Out/1 -> Scope/3
  Gateway Out5/1 -> Scope/4
  Gateway Out4/1 -> Scope/5
  Time Division Demultiplexer/1 -> Register/1
  Time Division Demultiplexer/2 -> Register1/1
  Time Division Demultiplexer/3 -> Register3/1
  Time Division Demultiplexer/4 -> Register4/1
  Time Division Demultiplexer/5 -> Register5/1
  Time Division Demultiplexer/6 -> Register6/1
  Time Division Demultiplexer/7 -> Register7/1
  Time Division Demultiplexer/8 -> Register8/1
  Time Division Demultiplexer/9 -> Register9/1
  Time Division Demultiplexer/10 -> Register10/1
  Time Division Demultiplexer/11 -> Register11/1
  Time Division Demultiplexer/12 -> Register12/1
  Time Division Demultiplexer1/1 -> Register16/1
  Time Division Demultiplexer1/2 -> Register17/1
  Time Division Demultiplexer1/3 -> Register18/1
  Time Division Demultiplexer1/4 -> Register13/1
  Time Division Demultiplexer1/5 -> Register14/1
  Time Division Demultiplexer1/6 -> Register15/1
  Time Division Demultiplexer1/7 -> Register22/1
  Time Division Demultiplexer1/8 -> Register23/1
  Time Division Demultiplexer1/9 -> Register24/1
  Time Division Demultiplexer1/10 -> Register19/1
  Time Division Demultiplexer1/11 -> Register20/1
  Time Division Demultiplexer1/12 -> Register21/1
  Register/1 -> [sin_ch1]
  Register1/1 -> [sin_ch2]
  Register3/1 -> [sin_ch3]
  Register5/1 -> [sin_ch5]
  Register4/1 -> [sin_ch4]
  Register6/1 -> [sin_ch6]
  Register12/1 -> [sin_ch12]
  Register8/1 -> [sin_ch8]
  Register9/1 -> [sin_ch9]
  Register11/1 -> [sin_ch11]
  Register7/1 -> [sin_ch7]
  Register10/1 -> [sin_ch10]
  Register16/1 -> [cos_ch1]
  Register13/1 -> [cos_ch4]
  Register18/1 -> [cos_ch3]
  Register14/1 -> [cos_ch5]
  Register15/1 -> [cos_ch6]
  Register17/1 -> [cos_ch2]
  Register19/1 -> [cos_ch10]
  Register20/1 -> [cos_ch11]
  Register24/1 -> [cos_ch9]
  Register22/1 -> [cos_ch7]
  Register23/1 -> [cos_ch8]
  Register21/1 -> [cos_ch12]
  [sin_ch1] -> Gateway Out3/1
  [cos_ch1] -> Gateway Out6/1
  Gateway Out3/1 -> Real-Imag to Complex/1
  Gateway Out6/1 -> Real-Imag to Complex/2
  "DDS Compiler 6.0 "/3 -> Time Division Demultiplexer/1
  "DDS Compiler 6.0 "/4 -> Time Division Demultiplexer1/1
  Real-Imag to Complex/1 -> Spectrum Analyzer/1
  Gateway Out7/1 -> Scope/6
  Gateway Out8/1 -> Scope/7
  "DDS Compiler 6.0 "/1 -> Gateway Out5/1
  "DDS Compiler 6.0 "/2 -> Gateway Out4/1
  "DDS Compiler 6.0 "/5 -> Gateway Out7/1
  "DDS Compiler 6.0 "/6 -> Gateway Out8/1
  Constant/1 -> "DDS Compiler 6.0 "/4
  Counter1/1 -> Relational1/1
  Constant1/1 -> Relational1/2
